simulink model "simulink_D6"  (R2016a)
settings: Solver=VariableStepAuto  StartTime=0.0  StopTime=70  RelTol=1e-3
values from neighbouring files (symbols this model uses):
  Ad = ssGd.A    [Simulacao_Rel_Est_com_Integrador.m]    (also in Simulador_Real_Estados_Discreto_Jesse_Alves.m = Pnd.A; auxiliar_simulink.m = [0.6163 0.1182 0.2366 -0.1182; 0.07238 0.369 0.02743 -0.1282; desafio6.m; desafio6_Octave.m)
  Bd = ssGd.B    [Simulacao_Rel_Est_com_Integrador.m]    (also in Simulador_Real_Estados_Discreto_Jesse_Alves.m = Pnd.B; auxiliar_simulink.m = [0.4814 7.113e-06; 0.3494 0.5722; 0.6988 0.1813; -0.3494 0.9; desafio6.m; desafio6_Octave.m)
  Cd = ssGd.C    [Simulacao_Rel_Est_com_Integrador.m]    (also in Simulador_Real_Estados_Discreto_Jesse_Alves.m = Pnd.C; auxiliar_simulink.m = [0.2613 0.01172 0.3434 -0.01172; 0.2222 0.01975 0.03949 0.28; desafio6.m; desafio6_Octave.m)
  Kd = [0.261403   0.051374   0.159841  -0.030382 ... (first row only)    [auxiliar_simulink.m]    (also in desafio6.m = place(Ad,Bd,polos); desafio6_Octave.m = place(Ad,Bd,polos))
  Ki = Ka(end-no+1:end,end-no+1:end)    [Simulacao_Rel_Est_com_Integrador.m]    (also in Simulador_Real_Estados_Discreto_Jesse_Alves.m = Ki; auxiliar_simulink.m = [0.3255  -0.1734; desafio6.m = Ka(:,n+1:n+q))
  ta = 2.07    [auxiliar_simulink.m]    (also in desafio6.m; desafio6_Octave.m)
settings Model: Creator=JesseAlves  LastModifiedBy=JesseAlves

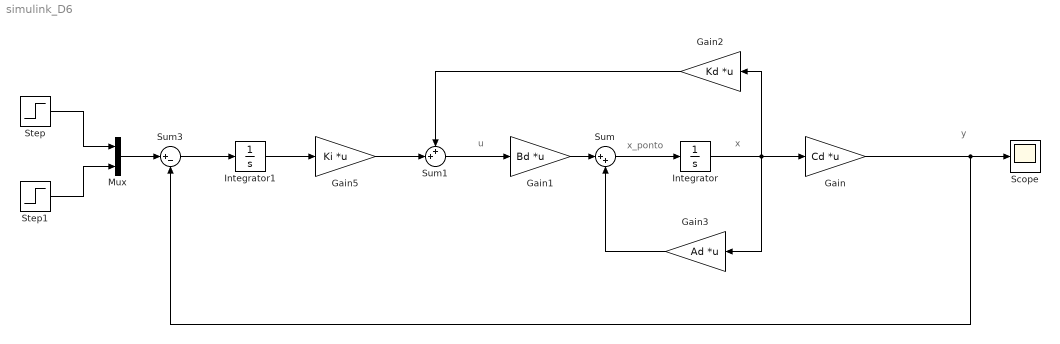
== system simulink_D6 ==
  note: y
  note: u
  note: x_ponto
  note: x
  Gain : Gain  Gain=Cd  Multiplication=Matrix(K*u)
  Gain1 : Gain  Gain=Bd  Multiplication=Matrix(K*u)
  Gain2 : Gain  Gain=Kd  Multiplication=Matrix(K*u)
  Gain3 : Gain  Gain=Ad  Multiplication=Matrix(K*u)
  Gain5 : Gain  Gain=Ki  Multiplication=Matrix(K*u)
  Integrator : Integrator
  Integrator1 : Integrator
  Mux : Mux  Inputs=2
  Scope : Scope
  Step : Step  Time=0  After=2  SampleTime=ta
  Step1 : Step  Time=0  SampleTime=ta
  Sum : Sum  Inputs=|++
  Sum1 : Sum  Inputs=++|
  Sum3 : Sum  Inputs=|+-
  wires:
  Integrator/1 -> Gain3/1, Gain2/1, Gain/1
  Gain1/1 -> Sum/1
  Sum1/1 -> Gain1/1
  Gain2/1 -> Sum1/1
  Gain3/1 -> Sum/2
  Gain/1 -> Scope/1, Sum3/2
  Step/1 -> Mux/1
  Step1/1 -> Mux/2
  Integrator1/1 -> Gain5/1
  Gain5/1 -> Sum1/2
  Mux/1 -> Sum3/1
  Sum3/1 -> Integrator1/1
  Sum/1 -> Integrator/1
